simulink model "PassStFtCtrl"  (R2024b)
settings: Solver=FixedStepDiscrete  StartTime=0.0  StopTime=10.0  FixedStep=0.01  RelTol=1e-3
undefined symbols (not defined in the file or in its folder): KeSMSuMdMotFinshdTm_Val, KeSMSuMdRetryTm1_Val, KeSMSuModeReqDurgTm_Val, KeSMSwPassStFtEnTrigBitMask_Val
libraries: StCtrlLib x1
settings Model: Creator=sn2xws  LastModifiedBy=sn55gm
settings SolverCC: AlgebraicLoopSolver=TrustRegion
settings DataIOCC: SaveFormat=StructureWithTime  ReturnWorkspaceOutputs=off
settings OptimizationCC: DefaultParameterBehavior=Inlined  EnhancedBackFolding=on  PassReuseOutputArgsAs=Individual arguments  ZeroExternalMemoryAtStartup=off  ZeroInternalMemoryAtStartup=off  OptimizeBlockOrder=speed  DifferentSizesBufferReuse=on  OptimizationCustomize=off  EfficientTunableParamExpr=on
settings DebuggingCC: ParameterTunabilityLossMsg=error  UnconnectedInputMsg=warning  UnconnectedOutputMsg=warning  UnconnectedLineMsg=warning  ArithmeticOperatorsInVariantConditions=warning
settings ModelReferenceCC: EnableRefExpFcnMdlSchedulingChecks=on  ModelReferenceNumInstancesAllowed=Single
settings SFSimCC: MATLABDynamicMemAlloc=off  CustomCodeUndefinedFunction=UseInterfaceOnly
settings RTWCC: Description=AUTOSAR  SystemTargetFile=autosar.tlc  GenCodeOnly=on  TemplateMakefile=ert_default_tmf  GenerateReport=on  IncludeHyperlinkInReport=on  LaunchReport=on  DataTypeReplacement=CDataTypesFixedWidth  GenerateTraceInfo=on  GenerateTraceReport=on  GenerateTraceReportSl=on  GenerateTraceReportSf=on  GenerateTraceReportEml=on  GenerateCodeMetricsReport=on  GPUComputeCapability=3.5
settings CodeAppCC: ForceParamTrailComments=on  IgnoreCustomStorageClasses=off  OperatorAnnotations=on  SimulinkDataObjDesc=on  SFDataObjDesc=on  InsertBlockDesc=on
settings STFCustomTargetCC: TargetLangStandard=C99 (ISO)  MultiwordLength=256  ParMdlRefBuildCompliant=on  CompOptLevelCompliant=on  IncludeMdlTerminateFcn=off  CombineOutputUpdateFcns=on  SuppressErrorStatus=on  ERTCustomFileBanners=on  SupportNonFinite=off  SupportComplex=off  SupportContinuousTime=off  SupportNonInlinedSFcns=off  RemoveResetFunc=on  MATLABClassNameForMDSCustomization=Simulink.SoftwareTarget.ERTCustomization  AutosarCompliant=on  UseToolchainInfoCompliant=on  LookupTableObjectStructAxisOrder=2,1,3,4,...  LUTObjectStructOrderEvenSpacing=Size,Table,Breakpoints  SystemTargetFile=autosar.tlc
settings ERTTargetCC: TargetLangStandard=C99 (ISO)  ConcurrentExecutionCompliant=off  IncludeMdlTerminateFcn=off  SuppressErrorStatus=on  SupportNonFinite=off  SupportComplex=off  ModelStepFunctionPrototypeControlCompliant=off  CPPClassGenCompliant=off  AutosarCompliant=on  LookupTableObjectStructAxisOrder=2,1,3,4,...  LUTObjectStructOrderEvenSpacing=Size,Table,Breakpoints  ERTCustomFileTemplate=example_file_process.tlc  ERTFilePackagingFormat=Compact  BooleanTrueId=TRUE  BooleanFalseId=FALSE  DynamicArrayContainerType=coder::array

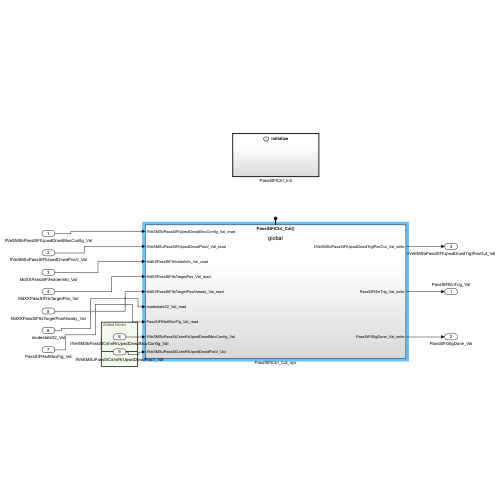
[thumbnail: Simulink's stored preview of the top-level diagram]
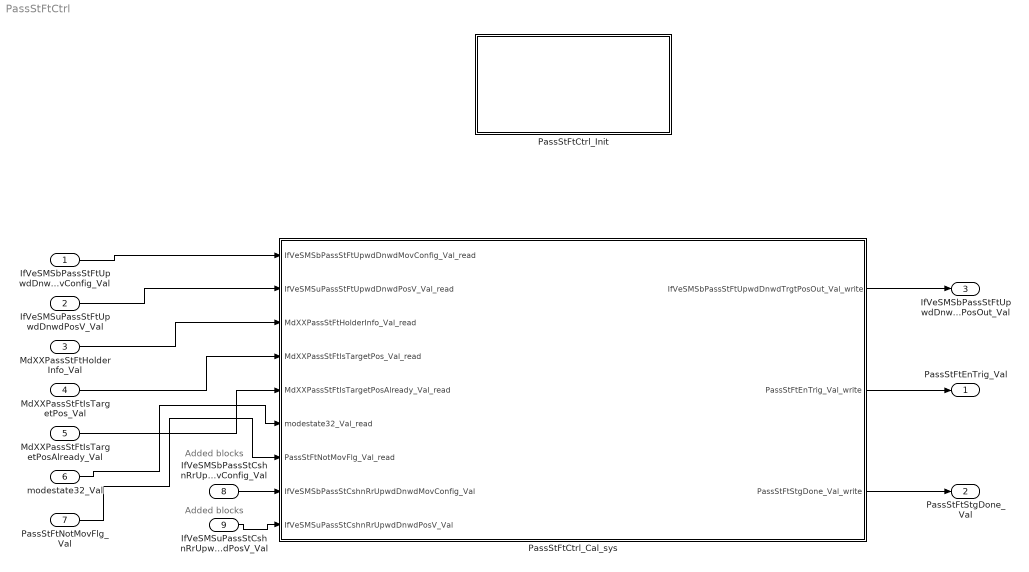
== system PassStFtCtrl ==
  note: Added blocks
  note: Added blocks
  IfVeSMSbPassStFtUpwdDnwdMovConfig_Val : Inport  OutDataTypeStr=boolean  PortDimensions=1
  IfVeSMSuPassStFtUpwdDnwdPosV_Val : Inport  Port=2  OutDataTypeStr=boolean  PortDimensions=1
  MdXXPassStFtHolderInfo_Val : Inport  Port=3  OutDataTypeStr=uint32  PortDimensions=1
  MdXXPassStFtIsTargetPos_Val : Inport  Port=4  OutDataTypeStr=uint32  PortDimensions=1
  MdXXPassStFtIsTargetPosAlready_Val : Inport  Port=5  OutDataTypeStr=uint32  PortDimensions=1
  modestate32_Val : Inport  Port=6  OutDataTypeStr=uint32  PortDimensions=1
  PassStFtNotMovFlg_Val : Inport  Port=7  OutDataTypeStr=boolean  PortDimensions=1
  IfVeSMSbPassStCshnRrUpwdDnwdMovConfig_Val : Inport  Port=8  OutDataTypeStr=boolean  PortDimensions=1
  IfVeSMSuPassStCshnRrUpwdDnwdPosV_Val : Inport  Port=9  OutDataTypeStr=boolean  PortDimensions=1
  PassStFtCtrl_Cal_sys : Subsystem
  PassStFtCtrl_Init : Subsystem
  PassStFtEnTrig_Val : Outport  OutDataTypeStr=boolean  PortDimensions=1  VectorParamsAs1DForOutWhenUnconnected=off
  PassStFtStgDone_Val : Outport  Port=2  OutDataTypeStr=boolean  PortDimensions=1  VectorParamsAs1DForOutWhenUnconnected=off
  IfVeSMSbPassStFtUpwdDnwdTrgtPosOut_Val : Outport  Port=3  OutDataTypeStr=boolean  PortDimensions=1  VectorParamsAs1DForOutWhenUnconnected=off
  wires:
  IfVeSMSbPassStFtUpwdDnwdMovConfig_Val/1 -> PassStFtCtrl_Cal_sys/1(IfVeSMSbPassStFtUpwdDnwdMovConfig_Val_read)
  IfVeSMSuPassStFtUpwdDnwdPosV_Val/1 -> PassStFtCtrl_Cal_sys/2(IfVeSMSuPassStFtUpwdDnwdPosV_Val_read)
  MdXXPassStFtHolderInfo_Val/1 -> PassStFtCtrl_Cal_sys/3(MdXXPassStFtHolderInfo_Val_read)
  MdXXPassStFtIsTargetPos_Val/1 -> PassStFtCtrl_Cal_sys/4(MdXXPassStFtIsTargetPos_Val_read)
  MdXXPassStFtIsTargetPosAlready_Val/1 -> PassStFtCtrl_Cal_sys/5(MdXXPassStFtIsTargetPosAlready_Val_read)
  modestate32_Val/1 -> PassStFtCtrl_Cal_sys/6(modestate32_Val_read)
  PassStFtNotMovFlg_Val/1 -> PassStFtCtrl_Cal_sys/7(PassStFtNotMovFlg_Val_read)
  PassStFtCtrl_Cal_sys/1(IfVeSMSbPassStFtUpwdDnwdTrgtPosOut_Val_write) -> IfVeSMSbPassStFtUpwdDnwdTrgtPosOut_Val/1
  PassStFtCtrl_Cal_sys/2(PassStFtEnTrig_Val_write) -> PassStFtEnTrig_Val/1
  PassStFtCtrl_Cal_sys/3(PassStFtStgDone_Val_write) -> PassStFtStgDone_Val/1
  IfVeSMSbPassStCshnRrUpwdDnwdMovConfig_Val/1 -> PassStFtCtrl_Cal_sys/8(IfVeSMSbPassStCshnRrUpwdDnwdMovConfig_Val)
  IfVeSMSuPassStCshnRrUpwdDnwdPosV_Val/1 -> PassStFtCtrl_Cal_sys/9(IfVeSMSuPassStCshnRrUpwdDnwdPosV_Val)

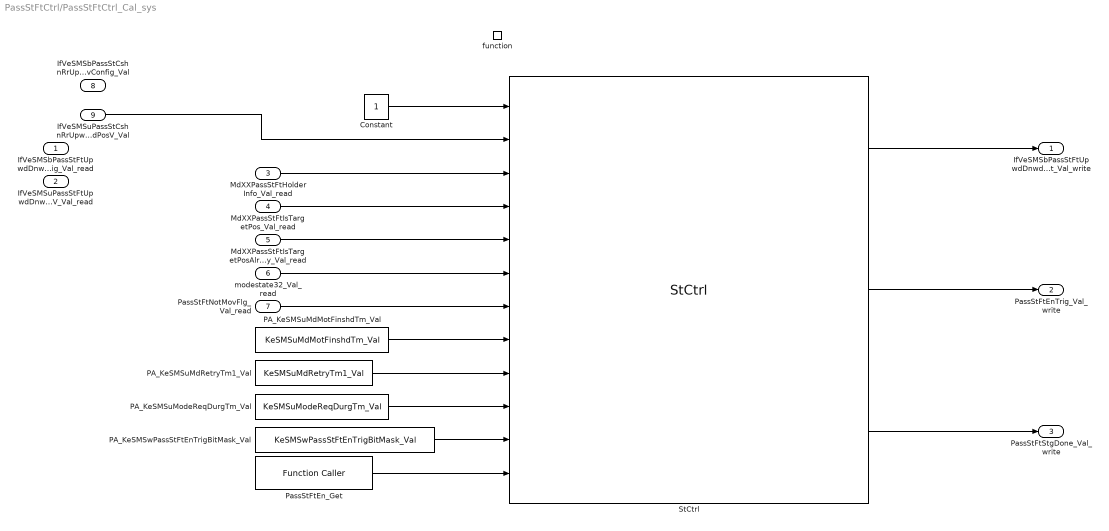
== system PassStFtCtrl/PassStFtCtrl_Cal_sys ==
  IfVeSMSbPassStFtUpwdDnwdMovConfig_Val_read : Inport
  IfVeSMSuPassStFtUpwdDnwdPosV_Val_read : Inport  Port=2
  MdXXPassStFtHolderInfo_Val_read : Inport  Port=3
  MdXXPassStFtIsTargetPos_Val_read : Inport  Port=4
  MdXXPassStFtIsTargetPosAlready_Val_read : Inport  Port=5
  modestate32_Val_read : Inport  Port=6
  PassStFtNotMovFlg_Val_read : Inport  Port=7
  IfVeSMSbPassStCshnRrUpwdDnwdMovConfig_Val : Inport  Port=8
  IfVeSMSuPassStCshnRrUpwdDnwdPosV_Val : Inport  Port=9
  function : TriggerPort  TriggerType=function-call  IsSimulinkFunction=on  FunctionName=PassStFtCtrl_Cal  VariantControl=(inherit)
  Constant : Constant  OutDataTypeStr=uint8
  PA_KeSMSuMdMotFinshdTm_Val : Constant  Value=KeSMSuMdMotFinshdTm_Val
  PA_KeSMSuMdRetryTm1_Val : Constant  Value=KeSMSuMdRetryTm1_Val
  PA_KeSMSuModeReqDurgTm_Val : Constant  Value=KeSMSuModeReqDurgTm_Val
  PA_KeSMSwPassStFtEnTrigBitMask_Val : Constant  Value=KeSMSwPassStFtEnTrigBitMask_Val
  PassStFtEn_Get : FunctionCaller  FunctionPrototype=data = PassStFtEn_Get()  InputArgumentSpecifications=<Enter example>  OutputArgumentSpecifications=uint32(1)
  StCtrl : StCtrlLib/StCtrl  SystemSampleTime=-1  VariantActivationTime=update diagram  AllowFlexibleInterface=on  Latency=0  AutoFrameSizeCalculation=off
  IfVeSMSbPassStFtUpwdDnwdTrgtPosOut_Val_write : Outport  VectorParamsAs1DForOutWhenUnconnected=off
      settings: EnsureOutportIsVirtual=on
  PassStFtEnTrig_Val_write : Outport  Port=2  VectorParamsAs1DForOutWhenUnconnected=off
      settings: EnsureOutportIsVirtual=on
  PassStFtStgDone_Val_write : Outport  Port=3  VectorParamsAs1DForOutWhenUnconnected=off
      settings: EnsureOutportIsVirtual=on
  wires:
  PA_KeSMSuMdMotFinshdTm_Val/1 -> StCtrl/8
  PA_KeSMSuMdRetryTm1_Val/1 -> StCtrl/9
  PA_KeSMSuModeReqDurgTm_Val/1 -> StCtrl/10
  PA_KeSMSwPassStFtEnTrigBitMask_Val/1 -> StCtrl/11
  PassStFtEn_Get/1 -> StCtrl/12
  StCtrl/1 -> IfVeSMSbPassStFtUpwdDnwdTrgtPosOut_Val_write/1
  StCtrl/2 -> PassStFtEnTrig_Val_write/1
  StCtrl/3 -> PassStFtStgDone_Val_write/1
  MdXXPassStFtHolderInfo_Val_read/1 -> StCtrl/3
  MdXXPassStFtIsTargetPos_Val_read/1 -> StCtrl/4
  MdXXPassStFtIsTargetPosAlready_Val_read/1 -> StCtrl/5
  modestate32_Val_read/1 -> StCtrl/6
  PassStFtNotMovFlg_Val_read/1 -> StCtrl/7
  IfVeSMSuPassStCshnRrUpwdDnwdPosV_Val/1 -> StCtrl/2
  Constant/1 -> StCtrl/1

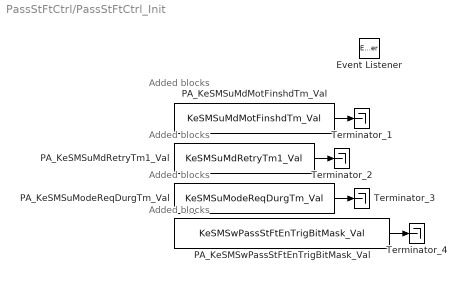
== system PassStFtCtrl/PassStFtCtrl_Init ==
  note: Added blocks
  note: Added blocks
  note: Added blocks
  note: Added blocks
  Event Listener : EventListener  EventName=reset
  PA_KeSMSuMdMotFinshdTm_Val : Constant  Value=KeSMSuMdMotFinshdTm_Val
  PA_KeSMSuMdRetryTm1_Val : Constant  Value=KeSMSuMdRetryTm1_Val
  PA_KeSMSuModeReqDurgTm_Val : Constant  Value=KeSMSuModeReqDurgTm_Val
  PA_KeSMSwPassStFtEnTrigBitMask_Val : Constant  Value=KeSMSwPassStFtEnTrigBitMask_Val
  Terminator_{1..4} (4 alike) : Terminator
  wires:
  PA_KeSMSuMdMotFinshdTm_Val/1 -> Terminator_1/1
  PA_KeSMSuMdRetryTm1_Val/1 -> Terminator_2/1
  PA_KeSMSuModeReqDurgTm_Val/1 -> Terminator_3/1
  PA_KeSMSwPassStFtEnTrigBitMask_Val/1 -> Terminator_4/1
